simulink model "Modellbildung_ParamEst"  (R2022a)
settings: Solver=VariableStepAuto  StartTime=0.0  StopTime=10.0  RelTol=1e-3
model workspace (MAT data in the model file):
  K = 1.1895
  T = 0.0910936537383
  TD = 0.65
settings Model: Creator=Uni  LastModifiedBy=Uni

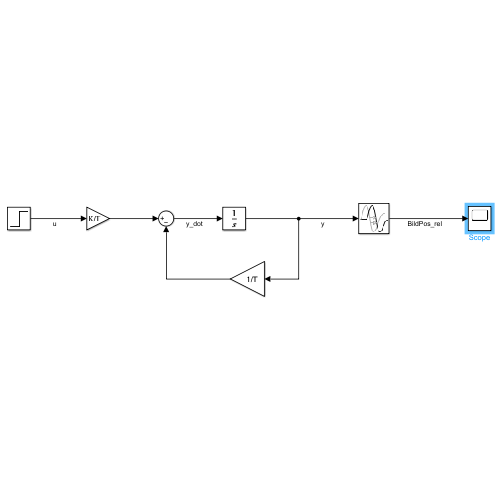
[thumbnail: Simulink's stored preview of the top-level diagram]
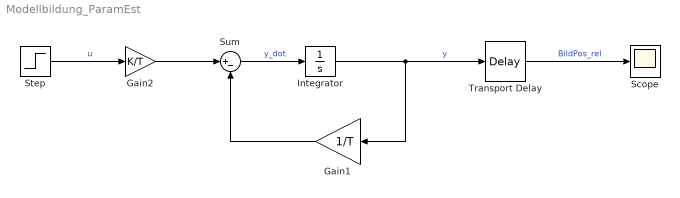
== system Modellbildung_ParamEst ==
  Gain1 : Gain  Gain=1/T
  Gain2 : Gain  Gain=K/T
  Integrator : Integrator
  Scope : Scope
  Step : Step  Time=0  Before=0.35  After=0.65  SampleTime=0
  Sum : Sum  Inputs=|+-
  Transport Delay : TransportDelay  DelayTime=TD
  wires:
  Step/1 -> Gain2/1  "u"
  Sum/1 -> Integrator/1  "y_dot"
  Integrator/1 -> Gain1/1, Transport Delay/1  "y"
  Gain1/1 -> Sum/2
  Gain2/1 -> Sum/1
  Transport Delay/1 -> Scope/1  "BildPos_rel"
